simulink model "SCM_PENDULUM_OKE"  (R2017b)
settings: Solver=FixedStepAuto  StartTime=0.0  StopTime=30  FixedStep=0.01  RelTol=1e-3
values from neighbouring files (symbols this model uses):
  n1 = par(bestchrom,1)    [GA.m]    (also in giatrin.m = 0.234; pidGA.m; tinhN.m = 0.171)
  n2 = par(bestchrom,2)    [GA.m]    (also in giatrin.m = 2.702; pidGA.m; tinhN.m = 1.596)
  n3 = par(bestchrom,3)    [GA.m]    (also in giatrin.m = 0.422; pidGA.m; tinhN.m = 0.307)
  n4 = par(bestchrom,4)    [GA.m]    (also in giatrin.m = 6.175; pidGA.m; tinhN.m = 1)
settings Model: Creator=DELL  LastModifiedBy=DELL

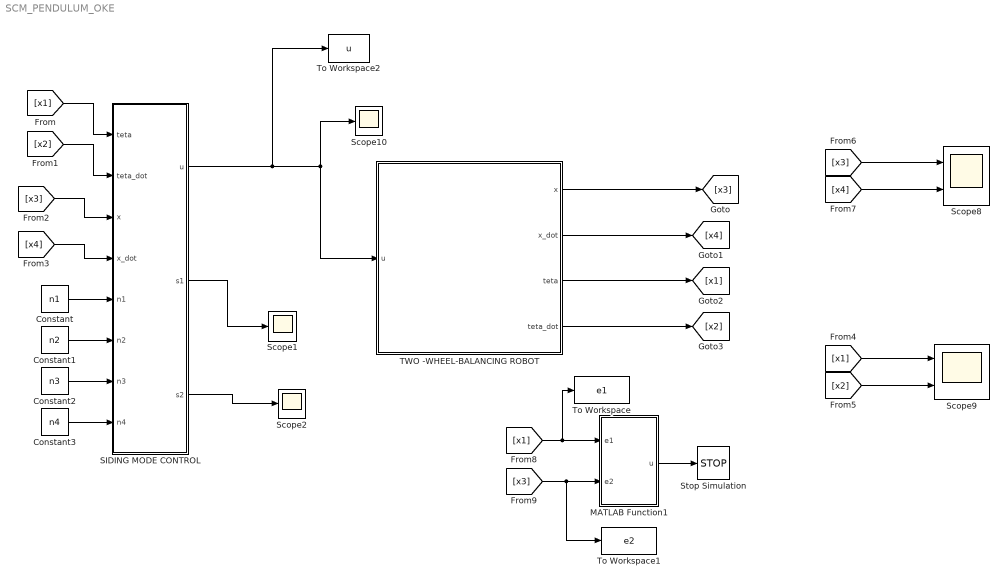
== system SCM_PENDULUM_OKE ==
  Constant : Constant  Value=n1
  Constant1 : Constant  Value=n2
  Constant2 : Constant  Value=n3
  Constant3 : Constant  Value=n4
  MATLAB Function1 : MATLAB Function  TreatAsAtomicUnit=on
  "SIDING MODE CONTROL " : MATLAB Function  TreatAsAtomicUnit=on
  Scope1 : Scope
  Scope10 : Scope
  Scope2 : Scope
  Scope8 : Scope  NumInputPorts=2
  Scope9 : Scope  NumInputPorts=2
  Stop Simulation : Stop
  TWO -WHEEL-BALANCING ROBOT : Subsystem
  To Workspace : ToWorkspace  VariableName=e1  SampleTime=-1
  To Workspace1 : ToWorkspace  VariableName=e2  SampleTime=-1
  To Workspace2 : ToWorkspace  VariableName=u  SampleTime=-1
  wires:
  "SIDING MODE CONTROL "/1(u) -> To Workspace2/1, TWO -WHEEL-BALANCING ROBOT/1(u), Scope10/1
  TWO -WHEEL-BALANCING ROBOT/1(x) -> [x3]
  TWO -WHEEL-BALANCING ROBOT/2(x_dot) -> [x4]
  TWO -WHEEL-BALANCING ROBOT/3(teta) -> [x1]
  TWO -WHEEL-BALANCING ROBOT/4(teta_dot) -> [x2]
  [x2] -> "SIDING MODE CONTROL "/2(teta_dot)
  [x1] -> "SIDING MODE CONTROL "/1(teta)
  [x3] -> "SIDING MODE CONTROL "/3(x)
  [x4] -> "SIDING MODE CONTROL "/4(x_dot)
  "SIDING MODE CONTROL "/2(s1) -> Scope1/1
  "SIDING MODE CONTROL "/3(s2) -> Scope2/1
  Constant/1 -> "SIDING MODE CONTROL "/5(n1)
  Constant1/1 -> "SIDING MODE CONTROL "/6(n2)
  Constant2/1 -> "SIDING MODE CONTROL "/7(n3)
  Constant3/1 -> "SIDING MODE CONTROL "/8(n4)
  MATLAB Function1/1(u) -> Stop Simulation/1
  [x1] -> To Workspace/1, MATLAB Function1/1(e1)
  [x3] -> To Workspace1/1, MATLAB Function1/2(e2)
  [x1] -> Scope9/1
  [x2] -> Scope9/2
  [x3] -> Scope8/1
  [x4] -> Scope8/2

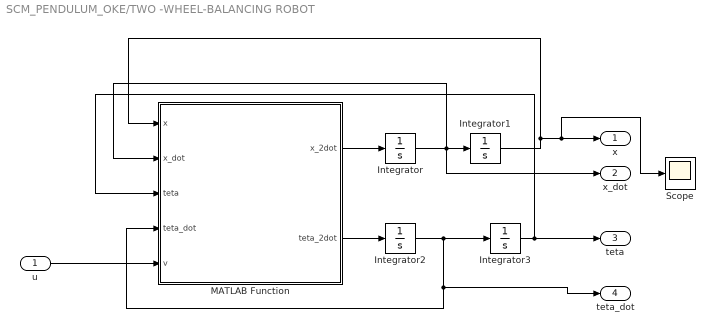
== system SCM_PENDULUM_OKE/TWO -WHEEL-BALANCING ROBOT ==
  u : Inport
  Integrator : Integrator
  Integrator1 : Integrator  InitialCondition=0.05
  Integrator2 : Integrator
  Integrator3 : Integrator  InitialCondition=0.05
  MATLAB Function : MATLAB Function  TreatAsAtomicUnit=on
  Scope : Scope
  x : Outport
  x_dot : Outport  Port=2
  teta : Outport  Port=3
  teta_dot : Outport  Port=4
  wires:
  Integrator2/1 -> teta_dot/1, MATLAB Function/4(teta_dot), Integrator3/1
  MATLAB Function/2(teta_2dot) -> Integrator2/1
  Integrator1/1 -> x/1, Scope/1, MATLAB Function/1(x)
  MATLAB Function/1(x_2dot) -> Integrator/1
  Integrator3/1 -> teta/1, MATLAB Function/3(teta)
  Integrator/1 -> x_dot/1, MATLAB Function/2(x_dot), Integrator1/1
  u/1 -> MATLAB Function/5(v)

== matlab function SCM_PENDULUM_OKE/TWO -WHEEL-BALANCING ROBOT/MATLAB Function ==
  data: x input; x_2dot output; x_dot input; teta input; teta_dot input; v input; teta_2dot output
function [x_2dot,teta_2dot] = fcn(x,x_dot,teta,teta_dot,v)
global v1 v2
g=9.81; %Gravity(m/s^2)
r=0.051; %Radius of wheel(m)
Mw=0.03; %Mass of wheel(kg)
Mp=1.13; %Mass of body(kg)
Iw=0.000039; %Inertia of the wheel(kg*m^2)
Ip=0.0041; %Inertia of the body(kg*m^2)
L=0.07; %Length to the body's center of mass(m)

%Motor's variables
Km=0.006123; %Motor torque constant(Nm/A)
Ke=0.006087; %Back EMF constant(Vs/rad)
R=3; %Nominal terminal resistance(Ohm)
a1=Mp*L/(Ip+Mp*L^2);
a2=Km*Ke/(R*r*(Ip+Mp*L^2));
a3=Km/(R*(Ip+Mp*L^2));
a4=Mp*g*L/(Ip+Mp*L^2);
b1=2*Km/(R*r*(2*Mw+2*(Iw/r^2)+Mp));
b2=2*Km*Ke/(R*r^2*(2*Mw+2*(Iw/r^2)+Mp));
b3=Mp*L/(2*Mw+2*(Iw/r^2)+Mp);
K=1.0e+03 *[-0.0316   -0.0361    1.6415    0.1272];


teta_2dot = -(a4*teta - 2*a3*v + 2*a2*x + a1*b1*v - a1*b2*x_dot)/(a1*b3 - 1);
x_2dot=-(b1*v - b2*x_dot + a4*b3*teta - 2*a3*b3*v + 2*a2*b3*x)/(a1*b3 - 1);

== matlab function SCM_PENDULUM_OKE/SIDING MODE CONTROL  ==
  data: u output; teta input; teta_dot input; s1 output; x input; x_dot input; s2 output; n1 input; n2 input; n3 input; n4 input
function [u,s1,s2]= SMC(teta,teta_dot,x,x_dot,n1,n2,n3,n4)

g=9.81; %Gravity(m/s^2)
r=0.051; %Radius of wheel(m)
Mw=0.03; %Mass of wheel(kg)
Mp=1.13; %Mass of body(kg)
Iw=0.000039; %Inertia of the wheel(kg*m^2)
Ip=0.0041; %Inertia of the body(kg*m^2)
L=0.07; %Length to the body's center of mass(m)
%landa=10;k1=20;k=2;
%Motor's variables
Km=0.006123; %Motor torque constant(Nm/A)
Ke=0.006087; %Back EMF constant(Vs/rad)
R=3; %Nominal terminal resistance(Ohm)
a1=Mp*L/(Ip+Mp*L^2);
a2=Km*Ke/(R*r*(Ip+Mp*L^2));
a3=Km/(R*(Ip+Mp*L^2));
a4=Mp*g*L/(Ip+Mp*L^2);
b1=2*Km/(R*r*(2*Mw+2*(Iw/r^2)+Mp));
b2=2*Km*Ke/(R*r^2*(2*Mw+2*(Iw/r^2)+Mp));
b3=Mp*L/(2*Mw+2*(Iw/r^2)+Mp);

g1=-(a1*b1- 2*a3)/(a1*b3 - 1);
f1=-(a4*teta + 2*a2*x  - a1*b2*x_dot)/(a1*b3 - 1);
g2=-(b1- 2*a3*b3)/(a1*b3 - 1);
f2=-(- b2*x_dot + a4*b3*teta + 2*a2*b3*x)/(a1*b3 - 1);
s1=teta+ n1*teta_dot;
s2=x+ n2*x_dot;
anpha= n1*sign(s1)*f1+ n3*sign(s2)*f2+teta_dot*sign(s1)+ n3*x_dot*sign(s2);
beta= n1*sign(s1)*g1+ n3*sign(s2)*g2;
u=(- n4-anpha)/beta;




%u2=1/g2*(yd_2d-landa*e2_d-f2-k1*s2-k*sign(s2));
%u1=1/g1*(yd_2d-landa*e1_d-f1-k1*s1-k*sign(s1));

== matlab function SCM_PENDULUM_OKE/MATLAB Function1 ==
  data: u output; e1 input; e2 input
function u = fcn(e1,e2)
if ((abs(e1)>2)||(abs(e2)>2))
    u=1;
else
    u=0;
end
